simulink model "ModelPrePostNear"  (R2022b)
settings: Solver=FixedStepDiscrete  StartTime=0.0  StopTime=1  RelTol=1e-3  EnableMultiTasking=on
InitFcn:
  | % Initialize model
  | run(['ModelInit.m']);
  | 
  | % load library data
  | GainLibrary_data;
StartFcn:
  | % make sure all the simulated RTC requests are found
  | %RTC_SIM_OBJ.ValidateREQs();
model workspace (MAT data in the model file):
  PreampVolumeTable_Idx = Simulink.Signal
  PreampVolumeTable_Idx.DataType = 'auto'
  PreampVolumeTable_Idx.Dimensions = -1
  PreampVolumeTable_Idx.DimensionsMode = 'auto'
  PreampVolumeTable_Idx.Complexity = 'auto'
  PreampVolumeTable_Idx.SampleTime = -1
  PreampVolumeTable_Idx.SamplingMode = 'auto'
  PreampVolumeTable_Idx.InitialValue = 'uint8([0 255 255 255 255 255])'
  Range = Simulink.Signal
  Range.DataType = 'auto'
  Range.Dimensions = -1
  Range.DimensionsMode = 'auto'
  Range.Complexity = 'auto'
  Range.SampleTime = -1
  Range.SamplingMode = 'auto'
  Table_Idx = Simulink.Signal
  Table_Idx.DataType = 'auto'
  Table_Idx.Dimensions = -1
  Table_Idx.DimensionsMode = 'auto'
  Table_Idx.Complexity = 'auto'
  Table_Idx.SampleTime = -1
  Table_Idx.SamplingMode = 'auto'
undefined symbols (not defined in the file): numAudioIn, preAmp, sys_defs
libraries: FeaturePath x11, RTC x6, SampleRateConverter x4, dspindex x3, EdgePorts x2, ToneBtc x2, dspsrcs4 x2, Router x1, Near1p1Ann x1, EnergyLimiter x1, Limiter x1, Mute x1
settings Model: Creator=kl13806  LastModifiedBy=sc48041
settings SolverCC: AlgebraicLoopSolver=TrustRegion  AutoInsertRateTranBlk=on
settings OptimizationCC: DefaultParameterBehavior=Inlined  DefaultUnderspecifiedDataType=single  EnhancedBackFolding=on  PassReuseOutputArgsAs=Individual arguments  ZeroExternalMemoryAtStartup=off  ZeroInternalMemoryAtStartup=off  MaxStackSize=2048  OptimizeBlockOrder=speed  DifferentSizesBufferReuse=on  OptimizationCustomize=off  EfficientTunableParamExpr=on
settings DebuggingCC: InheritedTsInSrcMsg=none  MultiTaskDSMMsg=none  MultiTaskRateTransMsg=warning  ParameterPrecisionLossMsg=none  ParameterTunabilityLossMsg=error  UnconnectedInputMsg=warning  UnconnectedOutputMsg=warning  UnconnectedLineMsg=warning  BusObjectLabelMismatch=none  UnknownTsInhSupMsg=none  SFUnexpectedBacktrackingDiag=warning  SFNoUnconditionalDefaultTransitionDiag=warning  SFExecutionAtInitializationDiag=none  SFMachineParentedDataDiag=warning  ArithmeticOperatorsInVariantConditions=warning
settings HardwareCC: ProdBitPerPointer=32  ProdBitPerSizeT=32  ProdBitPerPtrDiffT=32  ProdWordSize=32  ProdHWDeviceType=Intel->x86-32 (Windows32)  TargetBitPerPointer=64  TargetBitPerSizeT=64  TargetBitPerPtrDiffT=64  TargetLongLongMode=on  TargetIntDivRoundTo=Zero  TargetEndianess=LittleEndian  TargetWordSize=64  TargetHWDeviceType=MATLAB Host  ProdEqTarget=off
settings ModelReferenceCC: EnableRefExpFcnMdlSchedulingChecks=on
settings SFSimCC: SimUseLocalCustomCode=off  MATLABDynamicMemAlloc=off  CustomCodeUndefinedFunction=UseInterfaceOnly
settings RTWCC: Description=Embedded Coder (host-based shared library target)  SystemTargetFile=ert_shrlib.tlc  GenCodeOnly=on  TemplateMakefile=ert_default_tmf  GenerateReport=on  RetainRTWFile=on  RTWUseLocalCustomCode=off  Toolchain=LCC-win64 v2.4.1 | gmake (64-bit Windows)  IncludeHyperlinkInReport=on  LaunchReport=on  GenerateTraceInfo=on  GenerateTraceReport=on  GenerateTraceReportSl=on  GenerateTraceReportSf=on  GenerateTraceReportEml=on  GenerateCodeMetricsReport=on  GenerateCodeReplacementReport=on
settings CodeAppCC: ForceParamTrailComments=on  IgnoreCustomStorageClasses=off  MaxIdLength=61  OperatorAnnotations=on  SimulinkDataObjDesc=on  SFDataObjDesc=on  InsertBlockDesc=on
settings STFCustomTargetCC: TargetLangStandard=C99 (ISO)  MultiwordLength=256  GenerateSampleERTMain=on  ParMdlRefBuildCompliant=on  CompOptLevelCompliant=on  CombineOutputUpdateFcns=on  ERTCustomFileBanners=on  SupportContinuousTime=off  SupportNonInlinedSFcns=off  RemoveResetFunc=on  SupportVariableSizeSignals=on  MATLABClassNameForMDSCustomization=Simulink.SoftwareTarget.ERTCustomization  ModelStepFunctionPrototypeControlCompliant=on  UseToolchainInfoCompliant=on  SystemTargetFile=ert_shrlib.tlc
settings ERTTargetCC: TargetLangStandard=C99 (ISO)  GenerateSampleERTMain=on  ConcurrentExecutionCompliant=off  SupportVariableSizeSignals=on  CPPClassGenCompliant=off  InlinedParameterPlacement=NonHierarchical  ERTCustomFileTemplate=example_file_process.tlc
settings ConfigComp: CovMetricSettings=dw  CovSaveCumulativeToWorkspaceVar=on  CovSaveSingleToWorkspaceVar=on  CovExternalEMLEnable=off

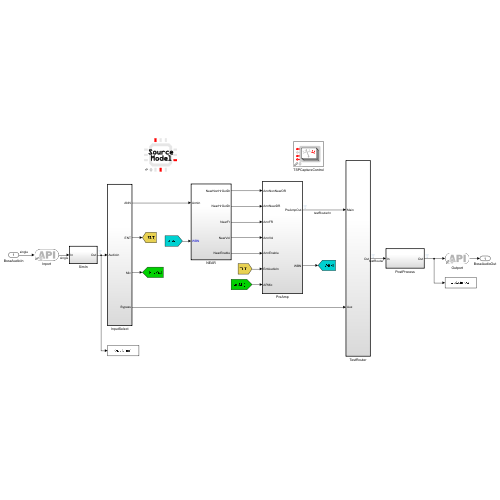
[thumbnail: Simulink's stored preview of the top-level diagram]
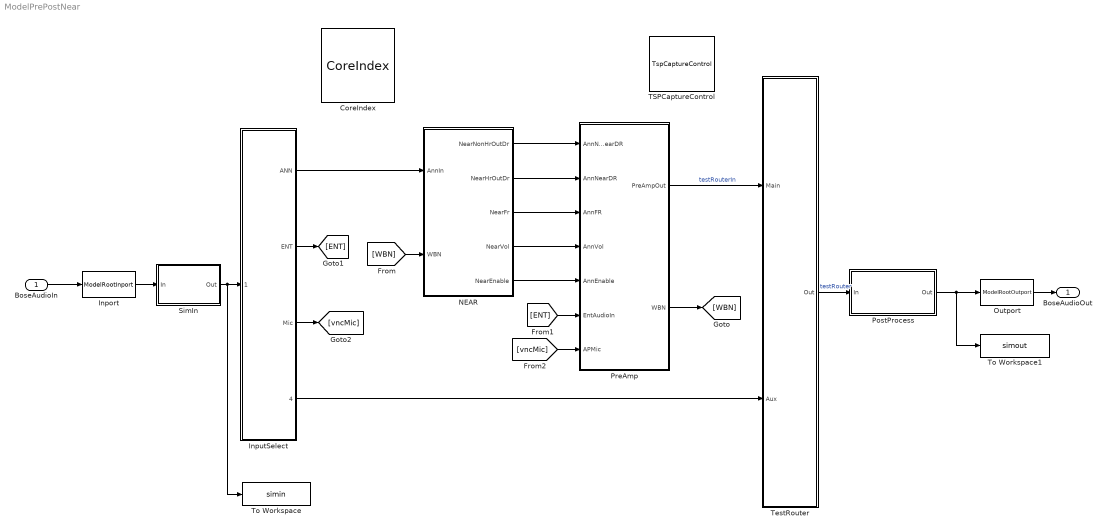
== system ModelPrePostNear ==
  BoseAudioIn : Inport  OutDataTypeStr=single  PortDimensions=[sys_defs.frameSize numAudioIn]  SampleTime=1/sys_defs.Fs * sys_defs.frameSize
  CoreIndex : FeaturePath/CoreIndex  Role=Source Model  CoreIndex=8  Config=[]  AddressingMode=Directly include core number in message identifiers (i.e. simple and static)  CrossCoreApi=None  CrossCoreAllocation=None  CrossCoreSampleTime=-1  BasePeriod=[]  TriggerInit=[-15 -776 80 -679]
      settings: SourceProductName=Bose Talaria
  Inport : EdgePorts/ModelRootInport  Config=ModelRootIn
      settings: SourceProductName=Bose Talaria
  InputSelect : Subsystem  TreatAsAtomicUnit=on
      settings: RTWSystemCode=Nonreusable function
  NEAR : Subsystem  TreatAsAtomicUnit=on
  Outport : EdgePorts/ModelRootOutport  Config=ModelRootOut
      settings: SourceProductName=Bose Talaria
  PostProcess : Subsystem  TreatAsAtomicUnit=on
  PreAmp : Subsystem  TreatAsAtomicUnit=on
  SimIn : Subsystem  TreatAsAtomicUnit=on
  TSPCaptureControl : TSP/TspCaptureControl  TriggerInit=[415 -766 500 -694]
      settings: SourceProductName=Bose Talaria
  TestRouter : Subsystem  TreatAsAtomicUnit=on
  To Workspace : ToWorkspace  VariableName=simin  SampleTime=-1
  To Workspace1 : ToWorkspace  VariableName=simout  SampleTime=-1
  BoseAudioOut : Outport  VectorParamsAs1DForOutWhenUnconnected=off
  wires:
  SimIn/1(Out) -> To Workspace/1, InputSelect/1(AudioIn)
  BoseAudioIn/1 -> Inport/1
  PostProcess/1(Out) -> To Workspace1/1, Outport/1
  TestRouter/1(Out) -> PostProcess/1(In)  "testRouter"
  PreAmp/1(PreAmpOut) -> TestRouter/1(Main)  "testRouterIn"
  InputSelect/4(Bypass) -> TestRouter/2(Aux)
  Inport/1 -> SimIn/1(In)
  Outport/1 -> BoseAudioOut/1
  InputSelect/1(ANN) -> NEAR/1(AnnIn)
  [WBN] -> NEAR/2(WBN)
  NEAR/5(NearEnable) -> PreAmp/5(AnnEnable)
  NEAR/4(NearVol) -> PreAmp/4(AnnVol)
  NEAR/3(NearFr) -> PreAmp/3(AnnFR)
  PreAmp/2(WBN) -> [WBN]
  NEAR/1(NearNonHrOutDr) -> PreAmp/1(AnnNonNearDR)
  NEAR/2(NearHrOutDr) -> PreAmp/2(AnnNearDR)
  InputSelect/2(ENT) -> [ENT]
  [ENT] -> PreAmp/6(EntAudioIn)
  InputSelect/3(Mic) -> [vncMic]
  [vncMic] -> PreAmp/7(APMic)

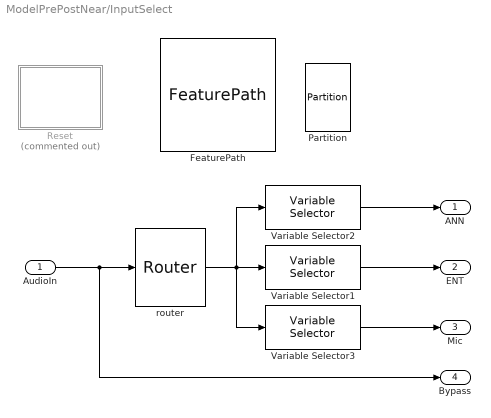
== system ModelPrePostNear/InputSelect ==
  AudioIn : Inport
  FeaturePath : FeaturePath/FeaturePath  FeatureName=InputSelect  IsGroup=on  GroupNumber=0  IsModule=on  TriggerInit=[105 216 220 329]
      settings: SourceProductName=Bose Talaria
  Partition : FeaturePath/Partition  PartitionNumber=0  TriggerInit=[250 241 295 309]
      settings: SourceProductName=Bose Talaria
  Reset : Subsystem  Commented=on
  Variable Selector1 : dspindex/Variable Selector  NumInputs=1  rowsOrCols=Columns  IdxMode=Fixed  Elements=entMap  ZerOneIdxMode=One-based  errmode=Clip Index  FillMode=on  FillValues=0
  Variable Selector2 : dspindex/Variable Selector  NumInputs=1  rowsOrCols=Columns  IdxMode=Fixed  Elements=annMap  ZerOneIdxMode=One-based  errmode=Clip Index  FillMode=on  FillValues=0
  Variable Selector3 : dspindex/Variable Selector  NumInputs=1  rowsOrCols=Columns  IdxMode=Fixed  Elements=vncMic  ZerOneIdxMode=One-based  errmode=Clip Index  FillMode=on  FillValues=0
  router : Router/Router  nInRouterMask=inputSelectChanIn  nOutRouterMask=inputSelectChanOut  outputMapDefaultRouterMask=inputSelectOutputMap
  ANN : Outport
  ENT : Outport  Port=2  VectorParamsAs1DForOutWhenUnconnected=off
  Mic : Outport  Port=3
  Bypass : Outport  Port=4  VectorParamsAs1DForOutWhenUnconnected=off
  wires:
  Variable Selector1/1 -> ENT/1
  AudioIn/1 -> Bypass/1, router/1
  router/1 -> Variable Selector3/1, Variable Selector2/1, Variable Selector1/1
  Variable Selector2/1 -> ANN/1
  Variable Selector3/1 -> Mic/1

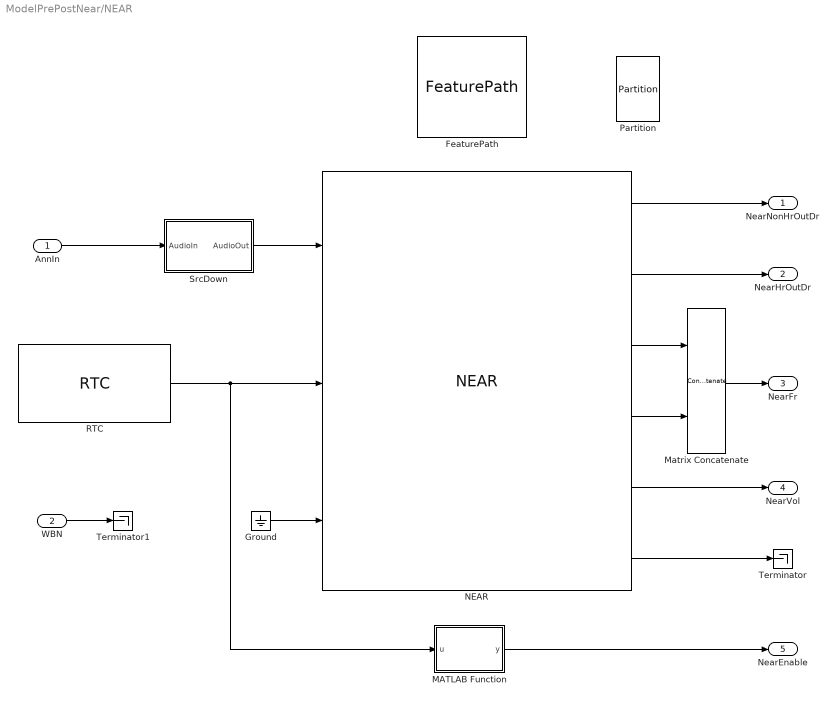
== system ModelPrePostNear/NEAR ==
  AnnIn : Inport
  WBN : Inport  Port=2
  FeaturePath : FeaturePath/FeaturePath  FeatureName=Near  IsGroup=on  GroupNumber=1  IsModule=on  TriggerInit=[15 -306 130 -199]
      settings: SourceProductName=Bose Talaria
  Ground : Ground
  MATLAB Function : MATLAB Function  TreatAsAtomicUnit=on
  Matrix Concatenate : Concatenate  Mode=Multidimensional array  ConcatenateDimension=2
  NEAR : Near1p1Ann/NEAR  near=near
  Partition : FeaturePath/Partition  PartitionNumber=0  TriggerInit=[225 -284 270 -216]
      settings: SourceProductName=Bose Talaria
  RTC : RTC/RTC  REQ_Priority=RTC_Mask.NormalPriority  RequestAtInit=off  EnableRequest=off  REQElemName1=Enable  REQElemType1=uint32  REQElemWidth1=1  REQElemInitial1=[0]  REQElemType2=uint32  REQElemWidth2=1  REQElemInitial2=[]  REQElemType3=uint32  REQElemWidth3=1  REQElemInitial3=[]  REQElemType4=uint32  REQElemWidth4=1  REQElemInitial4=[]  REQElemType5=uint32  REQElemWidth5=1  REQElemInitial5=[]  REQElemType6=uint32  REQElemWidth6=1  REQElemInitial6=[]  REQElemType7=uint32  REQElemWidth7=1  REQElemInitial7=[]  REQElemType8=uint32  REQElemWidth8=1  REQElemInitial8=[]  REQElemType9=uint32  REQElemWidth9=1  REQElemInitial9=[]  REQElemType10=uint32  REQElemWidth10=1  REQElemInitial10=[]  EnableResponse=on  EnableRSP_StatusIn=off  RSPElemType1=uint32  RSPElemWidth1=1  RSPElemType2=uint32  RSPElemWidth2=1  RSPElemType3=uint32  RSPElemWidth3=1  RSPElemType4=uint32  RSPElemWidth4=1  RSPElemType5=uint32  RSPElemWidth5=1  RSPElemType6=uint32  RSPElemWidth6=1  RSPElemType7=uint32  RSPElemWidth7=1  RSPElemType8=uint32  RSPElemWidth8=1  RSPElemType9=uint32  RSPElemWidth9=1  RSPElemType10=uint32  RSPElemWidth10=1  EnableNotification=off  EnableNTF_PrepTrig=off  NTFElemType1=uint32  NTFElemWidth1=1  NTFElemType2=uint32  NTFElemWidth2=1  NTFElemType3=uint32  NTFElemWidth3=1  NTFElemType4=uint32  NTFElemWidth4=1  NTFElemType5=uint32  NTFElemWidth5=1  NTFElemType6=uint32  NTFElemWidth6=1  NTFElemType7=uint32  NTFElemWidth7=1  NTFElemType8=uint32  NTFElemWidth8=1  NTFElemType9=uint32  NTFElemWidth9=1  NTFElemType10=uint32  NTFElemWidth10=1  MaskMessageName=Enable
      settings: SourceProductName=Bose Talaria
  SrcDown : Subsystem  TreatAsAtomicUnit=on
      settings: RTWSystemCode=Nonreusable function
  Terminator : Terminator
  Terminator1 : Terminator
  NearNonHrOutDr : Outport
  NearHrOutDr : Outport  Port=2
  NearFr : Outport  Port=3
  NearVol : Outport  Port=4
  NearEnable : Outport  Port=5
  wires:
  NEAR/1 -> NearNonHrOutDr/1
  AnnIn/1 -> SrcDown/1(AudioIn)
  NEAR/2 -> NearHrOutDr/1
  NEAR/3 -> Matrix Concatenate/1
  NEAR/4 -> Matrix Concatenate/2
  Matrix Concatenate/1 -> NearFr/1
  NEAR/5 -> NearVol/1
  NEAR/6 -> Terminator/1
  RTC/1 -> NEAR/2, MATLAB Function/1(u)
  MATLAB Function/1(y) -> NearEnable/1
  SrcDown/1(AudioOut) -> NEAR/1
  Ground/1 -> NEAR/3
  WBN/1 -> Terminator1/1

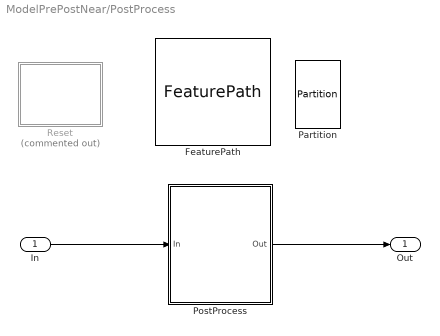
== system ModelPrePostNear/PostProcess ==
  In : Inport
  FeaturePath : FeaturePath/FeaturePath  FeatureName=PostProcess  IsGroup=on  GroupNumber=3  IsModule=on  TriggerInit=[85 -186 200 -79]
      settings: SourceProductName=Bose Talaria
  Partition : FeaturePath/Partition  PartitionNumber=0  TriggerInit=[225 -164 270 -96]
      settings: SourceProductName=Bose Talaria
  PostProcess : Subsystem  TreatAsAtomicUnit=on
      settings: RTWSystemCode=Nonreusable function  RTWFcnNameOpts=Use subsystem name  RTWFileNameOpts=Use subsystem name  FunctionWithSeparateData=on
  Reset : Subsystem  Commented=on
  Out : Outport  VectorParamsAs1DForOutWhenUnconnected=off
  wires:
  In/1 -> PostProcess/1(In)
  PostProcess/1(Out) -> Out/1

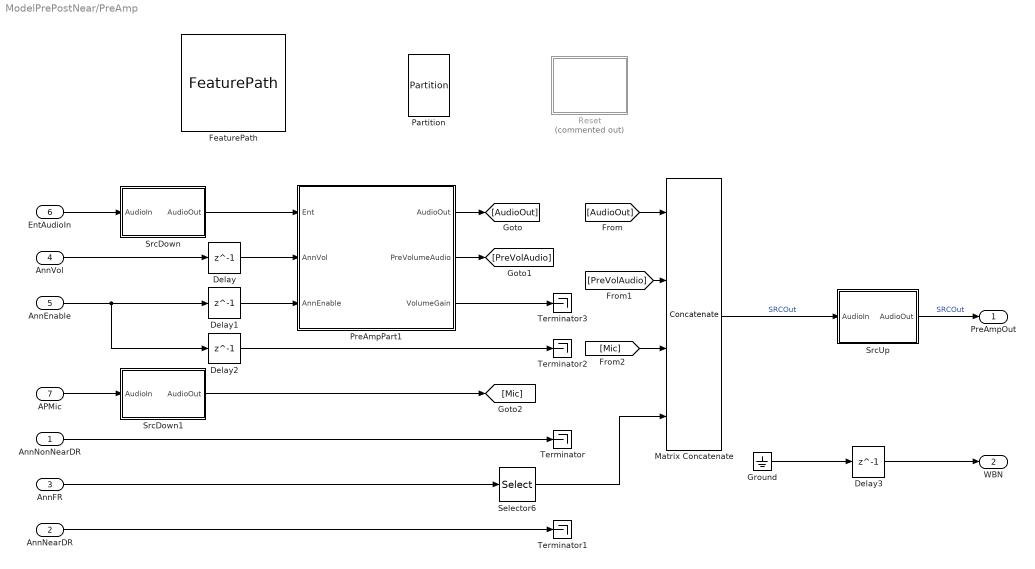
== system ModelPrePostNear/PreAmp ==
  AnnNonNearDR : Inport
  AnnNearDR : Inport  Port=2
  AnnFR : Inport  Port=3
  AnnVol : Inport  Port=4
  AnnEnable : Inport  Port=5
  EntAudioIn : Inport  Port=6
  APMic : Inport  Port=7
  Delay{,1..3} (4 alike) : Delay  DelayLength=1
  FeaturePath : FeaturePath/FeaturePath  FeatureName=PreAmp  IsGroup=on  GroupNumber=2  IsModule=on  TriggerInit=[-135 -246 -20 -139]
      settings: SourceProductName=Bose Talaria
  Ground : Ground
  Matrix Concatenate : Concatenate  NumInputs=4  Mode=Multidimensional array  ConcatenateDimension=2
  Partition : FeaturePath/Partition  PartitionNumber=0  TriggerInit=[115 -224 160 -156]
      settings: SourceProductName=Bose Talaria
  PreAmpPart1 : Subsystem  TreatAsAtomicUnit=on
      settings: RTWSystemCode=Nonreusable function
  Reset : Subsystem  Commented=on
  Selector6 : Selector  NumberOfDimensions=2  InputPortWidth=3  IndexOptions=Select all,Index vector (dialog)  Indices=4,1:19  OutputSizes=1,1
  SrcDown : Subsystem  TreatAsAtomicUnit=on
      settings: RTWSystemCode=Nonreusable function
  SrcDown1 : Subsystem  TreatAsAtomicUnit=on
      settings: RTWSystemCode=Nonreusable function
  SrcUp : Subsystem  TreatAsAtomicUnit=on
      settings: RTWSystemCode=Nonreusable function
  Terminator{,1..3} (4 alike) : Terminator
  PreAmpOut : Outport  VectorParamsAs1DForOutWhenUnconnected=off
  WBN : Outport  Port=2
  wires:
  EntAudioIn/1 -> SrcDown/1(AudioIn)
  Matrix Concatenate/1 -> SrcUp/1(AudioIn)  "SRCOut"
  SrcUp/1(AudioOut) -> PreAmpOut/1  "SRCOut"
  Delay3/1 -> WBN/1
  SrcDown/1(AudioOut) -> PreAmpPart1/1(Ent)
  AnnVol/1 -> Delay/1
  AnnEnable/1 -> Delay2/1, Delay1/1
  Delay/1 -> PreAmpPart1/2(AnnVol)
  Delay1/1 -> PreAmpPart1/3(AnnEnable)
  AnnNonNearDR/1 -> Terminator/1
  AnnNearDR/1 -> Terminator1/1
  AnnFR/1 -> Selector6/1
  APMic/1 -> SrcDown1/1(AudioIn)
  PreAmpPart1/3(VolumeGain) -> Terminator3/1
  Delay2/1 -> Terminator2/1
  Ground/1 -> Delay3/1
  SrcDown1/1(AudioOut) -> [Mic]
  PreAmpPart1/1(AudioOut) -> [AudioOut]
  PreAmpPart1/2(PreVolumeAudio) -> [PreVolAudio]
  [AudioOut] -> Matrix Concatenate/1
  [PreVolAudio] -> Matrix Concatenate/2
  [Mic] -> Matrix Concatenate/3
  Selector6/1 -> Matrix Concatenate/4

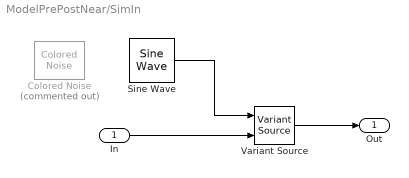
== system ModelPrePostNear/SimIn ==
  In : Inport  OutDataTypeStr=single  SampleTime=1/sys_defs.Fs * sys_defs.frameSize
  Colored Noise : dspsrcs4/Colored Noise  Commented=on  Color=pink  InverseFrequencyPower=1  BoundedOutput=on  NumChannels=2  OutputDataType=single  SamplesPerFrame=32  SampleTime=1/48000  RandomStream=mt19937ar with seed  Seed=67  SimulateUsing=Interpreted execution
  Sine Wave : dspsrcs4/Sine Wave  Amplitude=[0.99*ones(1,numAudioIn)]  Frequency=[150 225 200 275 325]  Phase=zeros(1,numAudioIn)  SampleMode=Discrete  OutComplex=Real  CompMethod=Trigonometric fcn  TableSize=Speed  SampleTime=1/sys_defs.Fs  SamplesPerFrame=sys_defs.frameSize  ResetState=Restart at time zero  OutputFrames=off  dataType=single  wordLen=16  udDataType=sfix(16)  fracBitsMode=Best precision  numFracBits=15  OutDataTypeStr=single  LastOutDataTypeStr=single
  Variant Source : VariantSource  VariantControlMode=sim codegen switching  ShowConditionOnBlock=on
  Out : Outport  VectorParamsAs1DForOutWhenUnconnected=off
  wires:
  In/1 -> Variant Source/2
  Variant Source/1 -> Out/1
  Sine Wave/1 -> Variant Source/1

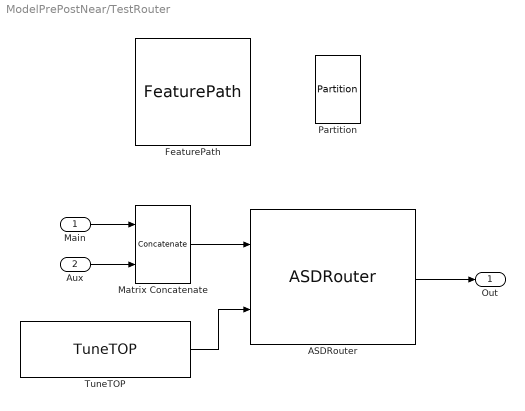
== system ModelPrePostNear/TestRouter ==
  Main : Inport
  Aux : Inport  Port=2
  ASDRouter : ASDRouter/ASDRouter  frameSize=sys_defs.frameSize  nChanOut=sys_defs.nAudioOut  mainSelect=main_select_test  numMainCh=num_main_chs  mainGain=main_gain_test  enableAux=enableAuxTestFlag  numAux=numAuxTestChannels  auxGain=aux_gain_test
  FeaturePath : FeaturePath/FeaturePath  FeatureName=TestRouter  IsGroup=on  GroupNumber=5  IsModule=off  TriggerInit=[290 -166 405 -59]
      settings: SourceProductName=Bose Talaria
  Matrix Concatenate : Concatenate  Mode=Multidimensional array  ConcatenateDimension=2
  Partition : FeaturePath/Partition  PartitionNumber=0  TriggerInit=[470 -149 515 -81]
      settings: SourceProductName=Bose Talaria
  TuneTOP : TuneVar/TuneTOP  TriggerInit=[175 117 345 173]  TopName=AuxSelect  TuneName=AuxSelect  DataType=int32  TunabilityNumber=1  MinValue=[]  MaxValue=[]  BankNumber=0  PreOverlay=false  PostOverlay=false  UseSameName=on  MaskValue=aux_select_test
      settings: SourceProductName=Bose Talaria
  Out : Outport
  wires:
  ASDRouter/1 -> Out/1
  TuneTOP/1 -> ASDRouter/2
  Matrix Concatenate/1 -> ASDRouter/1
  Main/1 -> Matrix Concatenate/1
  Aux/1 -> Matrix Concatenate/2

== system ModelPrePostNear/InputSelect/Reset ==
  MATLAB Function : MATLAB Function  TreatAsAtomicUnit=on
  RTC : RTC/RTC  REQ_Priority=RTC_Mask.NormalPriority  RequestAtInit=off  EnableRequest=on  REQElemType1=uint32  REQElemWidth1=1  REQElemInitial1=[]  REQElemType2=uint32  REQElemWidth2=1  REQElemInitial2=[]  REQElemType3=uint32  REQElemWidth3=1  REQElemInitial3=[]  REQElemType4=uint32  REQElemWidth4=1  REQElemInitial4=[]  REQElemType5=uint32  REQElemWidth5=1  REQElemInitial5=[]  REQElemType6=uint32  REQElemWidth6=1  REQElemInitial6=[]  REQElemType7=uint32  REQElemWidth7=1  REQElemInitial7=[]  REQElemType8=uint32  REQElemWidth8=1  REQElemInitial8=[]  REQElemType9=uint32  REQElemWidth9=1  REQElemInitial9=[]  REQElemType10=uint32  REQElemWidth10=1  REQElemInitial10=[]  EnableResponse=on  EnableRSP_StatusIn=off  RSPElemType1=uint32  RSPElemWidth1=1  RSPElemType2=uint32  RSPElemWidth2=1  RSPElemType3=uint32  RSPElemWidth3=1  RSPElemType4=uint32  RSPElemWidth4=1  RSPElemType5=uint32  RSPElemWidth5=1  RSPElemType6=uint32  RSPElemWidth6=1  RSPElemType7=uint32  RSPElemWidth7=1  RSPElemType8=uint32  RSPElemWidth8=1  RSPElemType9=uint32  RSPElemWidth9=1  RSPElemType10=uint32  RSPElemWidth10=1  EnableNotification=off  EnableNTF_PrepTrig=off  NTFElemType1=uint32  NTFElemWidth1=1  NTFElemType2=uint32  NTFElemWidth2=1  NTFElemType3=uint32  NTFElemWidth3=1  NTFElemType4=uint32  NTFElemWidth4=1  NTFElemType5=uint32  NTFElemWidth5=1  NTFElemType6=uint32  NTFElemWidth6=1  NTFElemType7=uint32  NTFElemWidth7=1  NTFElemType8=uint32  NTFElemWidth8=1  NTFElemType9=uint32  NTFElemWidth9=1  NTFElemType10=uint32  NTFElemWidth10=1  MaskMessageName=Reset
      settings: SourceProductName=Bose Talaria
  wires:
  RTC/1 -> MATLAB Function/Trigger

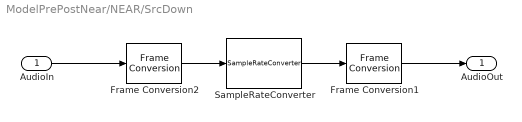
== system ModelPrePostNear/NEAR/SrcDown ==
  AudioIn : Inport
  Frame Conversion1 : FrameConversion  OutFrame=Sample-based
  Frame Conversion2 : FrameConversion
  SampleRateConverter : SampleRateConverter/SampleRateConverter  UPFACTOR=12  DOWNFACTOR=13  OUTFRAME_SIZE=-1  RATE_SELECTOR=Input Sample Rate  FS=48000  FPASSBAND=16500  FHEARING=19000  PASSBAND_RIPPLE=60  STOPBAND_ATTENUATION=60
  AudioOut : Outport
  wires:
  SampleRateConverter/1 -> Frame Conversion1/1
  AudioIn/1 -> Frame Conversion2/1
  Frame Conversion1/1 -> AudioOut/1
  Frame Conversion2/1 -> SampleRateConverter/1

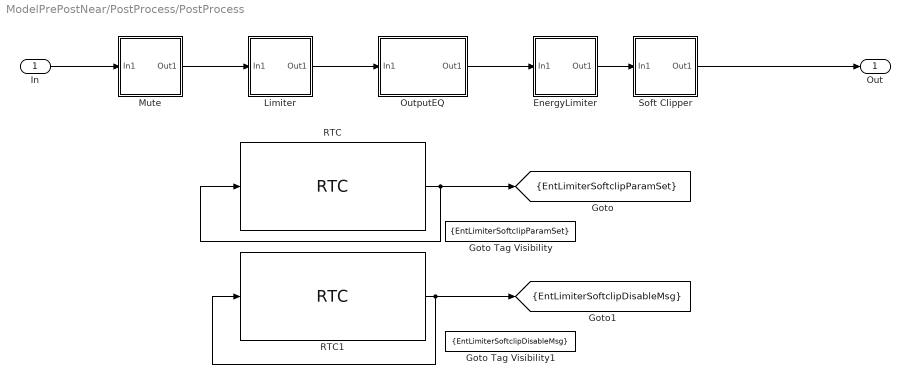
== system ModelPrePostNear/PostProcess/PostProcess ==
  In : Inport
  EnergyLimiter : Subsystem
  Goto Tag Visibility : GotoTagVisibility  GotoTag=EntLimiterSoftclipParamSet
  Goto Tag Visibility1 : GotoTagVisibility  GotoTag=EntLimiterSoftclipDisableMsg
  Limiter : Subsystem
  Mute : Subsystem
  OutputEQ : Subsystem
  RTC : RTC/RTC  Description=|  REQ_Priority=RTC_Mask.NormalPriority  RequestAtInit=off  EnableRequest=off  REQElemName1=paramSet  REQElemType1=uint32  REQElemWidth1=1  REQElemInitial1=1  REQElemType2=uint32  REQElemWidth2=1  REQElemInitial2=[]  REQElemType3=uint32  REQElemWidth3=1  REQElemInitial3=[]  REQElemType4=uint32  REQElemWidth4=1  REQElemInitial4=[]  REQElemType5=uint32  REQElemWidth5=1  REQElemInitial5=[]  REQElemType6=uint32  REQElemWidth6=1  REQElemInitial6=[]  REQElemType7=uint32  REQElemWidth7=1  REQElemInitial7=[]  REQElemType8=uint32  REQElemWidth8=1  REQElemInitial8=[]  REQElemType9=uint32  REQElemWidth9=1  REQElemInitial9=[]  REQElemType10=uint32  REQElemWidth10=1  REQElemInitial10=[]  EnableResponse=on  EnableRSP_StatusIn=off  RSPElemName1=paramSet  RSPElemType1=uint32  RSPElemWidth1=1  RSPElemType2=uint32  RSPElemWidth2=1  RSPElemType3=uint32  RSPElemWidth3=1  RSPElemType4=uint32  RSPElemWidth4=1  RSPElemType5=uint32  RSPElemWidth5=1  RSPElemType6=uint32  RSPElemWidth6=1  RSPElemType7=uint32  RSPElemWidth7=1  RSPElemType8=uint32  RSPElemWidth8=1  RSPElemType9=uint32  RSPElemWidth9=1  RSPElemType10=uint32  RSPElemWidth10=1  EnableNotification=off  EnableNTF_PrepTrig=off  NTFElemType1=uint32  NTFElemWidth1=1  NTFElemType2=uint32  NTFElemWidth2=1  NTFElemType3=uint32  NTFElemWidth3=1  NTFElemType4=uint32  NTFElemWidth4=1  NTFElemType5=uint32  NTFElemWidth5=1  NTFElemType6=uint32  NTFElemWidth6=1  NTFElemType7=uint32  NTFElemWidth7=1  NTFElemType8=uint32  NTFElemWidth8=1  NTFElemType9=uint32  NTFElemWidth9=1  NTFElemType10=uint32  NTFElemWidth10=1  MaskMessageName=LimiterSoftclipParamSet
      | Choose parameter set for limiter and soft clipper.
      | 1: normal set
      | 2: used in start-stop situation
      settings: SourceProductName=Bose Talaria
  RTC1 : RTC/RTC  REQ_Priority=RTC_Mask.NormalPriority  RequestAtInit=off  EnableRequest=off  REQElemName1=disableMsg  REQElemType1=uint32  REQElemWidth1=1  REQElemInitial1=0  REQElemType2=uint32  REQElemWidth2=1  REQElemInitial2=[]  REQElemType3=uint32  REQElemWidth3=1  REQElemInitial3=[]  REQElemType4=uint32  REQElemWidth4=1  REQElemInitial4=[]  REQElemType5=uint32  REQElemWidth5=1  REQElemInitial5=[]  REQElemType6=uint32  REQElemWidth6=1  REQElemInitial6=[]  REQElemType7=uint32  REQElemWidth7=1  REQElemInitial7=[]  REQElemType8=uint32  REQElemWidth8=1  REQElemInitial8=[]  REQElemType9=uint32  REQElemWidth9=1  REQElemInitial9=[]  REQElemType10=uint32  REQElemWidth10=1  REQElemInitial10=[]  EnableResponse=on  EnableRSP_StatusIn=off  RSPElemName1=disableMsg  RSPElemType1=uint32  RSPElemWidth1=1  RSPElemType2=uint32  RSPElemWidth2=1  RSPElemType3=uint32  RSPElemWidth3=1  RSPElemType4=uint32  RSPElemWidth4=1  RSPElemType5=uint32  RSPElemWidth5=1  RSPElemType6=uint32  RSPElemWidth6=1  RSPElemType7=uint32  RSPElemWidth7=1  RSPElemType8=uint32  RSPElemWidth8=1  RSPElemType9=uint32  RSPElemWidth9=1  RSPElemType10=uint32  RSPElemWidth10=1  EnableNotification=off  EnableNTF_PrepTrig=off  NTFElemType1=uint32  NTFElemWidth1=1  NTFElemType2=uint32  NTFElemWidth2=1  NTFElemType3=uint32  NTFElemWidth3=1  NTFElemType4=uint32  NTFElemWidth4=1  NTFElemType5=uint32  NTFElemWidth5=1  NTFElemType6=uint32  NTFElemWidth6=1  NTFElemType7=uint32  NTFElemWidth7=1  NTFElemType8=uint32  NTFElemWidth8=1  NTFElemType9=uint32  NTFElemWidth9=1  NTFElemType10=uint32  NTFElemWidth10=1  MaskMessageName=LimiterSoftclipDisable
      settings: SourceProductName=Bose Talaria
  Soft Clipper : Subsystem
  Out : Outport  VectorParamsAs1DForOutWhenUnconnected=off
  tag scope: EntLimiterSoftclipDisableMsg=scoped, EntLimiterSoftclipParamSet=scoped
  wires:
  Mute/1(Out1) -> Limiter/1(In1)
  Limiter/1(Out1) -> OutputEQ/1(In1)
  In/1 -> Mute/1(In1)
  OutputEQ/1(Out1) -> EnergyLimiter/1(In1)
  EnergyLimiter/1(Out1) -> Soft Clipper/1(In1)
  RTC1/1 -> RTC1/1, [EntLimiterSoftclipDisableMsg]
  RTC/1 -> RTC/1, [EntLimiterSoftclipParamSet]
  Soft Clipper/1(Out1) -> Out/1

== system ModelPrePostNear/PostProcess/Reset ==
  MATLAB Function : MATLAB Function  TreatAsAtomicUnit=on
  RTC : RTC/RTC  REQ_Priority=RTC_Mask.NormalPriority  RequestAtInit=off  EnableRequest=on  REQElemType1=uint32  REQElemWidth1=1  REQElemInitial1=[]  REQElemType2=uint32  REQElemWidth2=1  REQElemInitial2=[]  REQElemType3=uint32  REQElemWidth3=1  REQElemInitial3=[]  REQElemType4=uint32  REQElemWidth4=1  REQElemInitial4=[]  REQElemType5=uint32  REQElemWidth5=1  REQElemInitial5=[]  REQElemType6=uint32  REQElemWidth6=1  REQElemInitial6=[]  REQElemType7=uint32  REQElemWidth7=1  REQElemInitial7=[]  REQElemType8=uint32  REQElemWidth8=1  REQElemInitial8=[]  REQElemType9=uint32  REQElemWidth9=1  REQElemInitial9=[]  REQElemType10=uint32  REQElemWidth10=1  REQElemInitial10=[]  EnableResponse=on  EnableRSP_StatusIn=off  RSPElemType1=uint32  RSPElemWidth1=1  RSPElemType2=uint32  RSPElemWidth2=1  RSPElemType3=uint32  RSPElemWidth3=1  RSPElemType4=uint32  RSPElemWidth4=1  RSPElemType5=uint32  RSPElemWidth5=1  RSPElemType6=uint32  RSPElemWidth6=1  RSPElemType7=uint32  RSPElemWidth7=1  RSPElemType8=uint32  RSPElemWidth8=1  RSPElemType9=uint32  RSPElemWidth9=1  RSPElemType10=uint32  RSPElemWidth10=1  EnableNotification=off  EnableNTF_PrepTrig=off  NTFElemType1=uint32  NTFElemWidth1=1  NTFElemType2=uint32  NTFElemWidth2=1  NTFElemType3=uint32  NTFElemWidth3=1  NTFElemType4=uint32  NTFElemWidth4=1  NTFElemType5=uint32  NTFElemWidth5=1  NTFElemType6=uint32  NTFElemWidth6=1  NTFElemType7=uint32  NTFElemWidth7=1  NTFElemType8=uint32  NTFElemWidth8=1  NTFElemType9=uint32  NTFElemWidth9=1  NTFElemType10=uint32  NTFElemWidth10=1  MaskMessageName=Reset
      settings: SourceProductName=Bose Talaria
  wires:
  RTC/1 -> MATLAB Function/Trigger

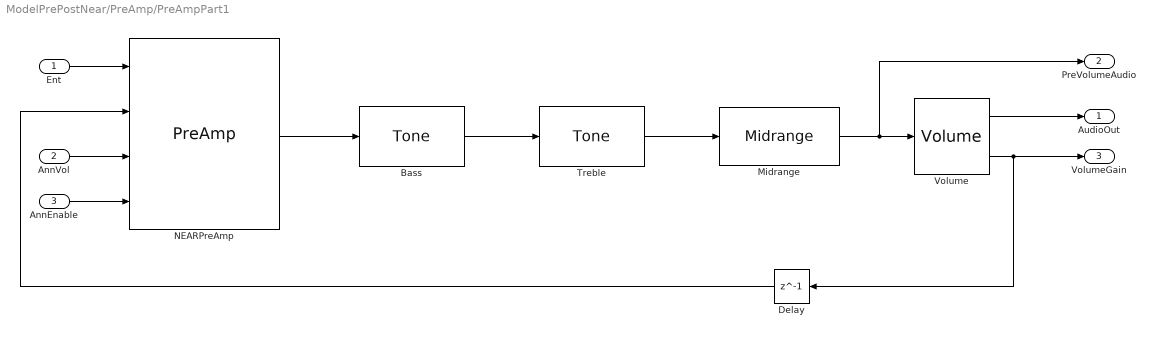
== system ModelPrePostNear/PreAmp/PreAmpPart1 ==
  Ent : Inport
  AnnVol : Inport  Port=2
  AnnEnable : Inport  Port=3
  Bass : ToneBtc/Tone  FeatureName=Bass  Config=[]  TriggerInit=[215 80 320 140]
      settings: SourceProductName=Bose Blocklib
  Delay : Delay  DelayLength=1
  Midrange : MidrangeBtc/Midrange  FeatureName=Midrange  Config=[]
      settings: SourceProductName=Bose Blocklib
  NEARPreAmp : PreAmpLib/PreAmp  Config=[preAmp]
  Treble : ToneBtc/Tone  FeatureName=Treble  Config=[]  TriggerInit=[395 80 500 140]
      settings: SourceProductName=Bose Blocklib
  Volume : VolumeBtc/Volume  FeatureName=Volume  Config=Volume  EnableGainOut=on  TriggerInit=[770 72 845 148]
      settings: SourceProductName=Bose Blocklib
  AudioOut : Outport
  PreVolumeAudio : Outport  Port=2
  VolumeGain : Outport  Port=3
  wires:
  Ent/1 -> NEARPreAmp/1
  Bass/1 -> Treble/1
  Treble/1 -> Midrange/1
  Midrange/1 -> PreVolumeAudio/1, Volume/1
  Volume/1 -> AudioOut/1
  Volume/2 -> Delay/1, VolumeGain/1
  NEARPreAmp/1 -> Bass/1
  Delay/1 -> NEARPreAmp/2
  AnnVol/1 -> NEARPreAmp/3
  AnnEnable/1 -> NEARPreAmp/4

== system ModelPrePostNear/PreAmp/Reset ==
  MATLAB Function : MATLAB Function  TreatAsAtomicUnit=on
  RTC : RTC/RTC  REQ_Priority=RTC_Mask.NormalPriority  RequestAtInit=off  EnableRequest=on  REQElemType1=uint32  REQElemWidth1=1  REQElemInitial1=[]  REQElemType2=uint32  REQElemWidth2=1  REQElemInitial2=[]  REQElemType3=uint32  REQElemWidth3=1  REQElemInitial3=[]  REQElemType4=uint32  REQElemWidth4=1  REQElemInitial4=[]  REQElemType5=uint32  REQElemWidth5=1  REQElemInitial5=[]  REQElemType6=uint32  REQElemWidth6=1  REQElemInitial6=[]  REQElemType7=uint32  REQElemWidth7=1  REQElemInitial7=[]  REQElemType8=uint32  REQElemWidth8=1  REQElemInitial8=[]  REQElemType9=uint32  REQElemWidth9=1  REQElemInitial9=[]  REQElemType10=uint32  REQElemWidth10=1  REQElemInitial10=[]  EnableResponse=on  EnableRSP_StatusIn=off  RSPElemType1=uint32  RSPElemWidth1=1  RSPElemType2=uint32  RSPElemWidth2=1  RSPElemType3=uint32  RSPElemWidth3=1  RSPElemType4=uint32  RSPElemWidth4=1  RSPElemType5=uint32  RSPElemWidth5=1  RSPElemType6=uint32  RSPElemWidth6=1  RSPElemType7=uint32  RSPElemWidth7=1  RSPElemType8=uint32  RSPElemWidth8=1  RSPElemType9=uint32  RSPElemWidth9=1  RSPElemType10=uint32  RSPElemWidth10=1  EnableNotification=off  EnableNTF_PrepTrig=off  NTFElemType1=uint32  NTFElemWidth1=1  NTFElemType2=uint32  NTFElemWidth2=1  NTFElemType3=uint32  NTFElemWidth3=1  NTFElemType4=uint32  NTFElemWidth4=1  NTFElemType5=uint32  NTFElemWidth5=1  NTFElemType6=uint32  NTFElemWidth6=1  NTFElemType7=uint32  NTFElemWidth7=1  NTFElemType8=uint32  NTFElemWidth8=1  NTFElemType9=uint32  NTFElemWidth9=1  NTFElemType10=uint32  NTFElemWidth10=1  MaskMessageName=Reset
      settings: SourceProductName=Bose Talaria
  wires:
  RTC/1 -> MATLAB Function/Trigger

== system ModelPrePostNear/PreAmp/SrcDown ==
  AudioIn : Inport
  Frame Conversion1 : FrameConversion  OutFrame=Sample-based
  Frame Conversion2 : FrameConversion
  SampleRateConverter : SampleRateConverter/SampleRateConverter  UPFACTOR=12  DOWNFACTOR=13  OUTFRAME_SIZE=-1  RATE_SELECTOR=Input Sample Rate  FS=48000  FPASSBAND=16500  FHEARING=19000  PASSBAND_RIPPLE=60  STOPBAND_ATTENUATION=60
  AudioOut : Outport
  wires:
  SampleRateConverter/1 -> Frame Conversion1/1
  AudioIn/1 -> Frame Conversion2/1
  Frame Conversion1/1 -> AudioOut/1
  Frame Conversion2/1 -> SampleRateConverter/1

== system ModelPrePostNear/PreAmp/SrcDown1 ==
  AudioIn : Inport
  Frame Conversion1 : FrameConversion  OutFrame=Sample-based
  Frame Conversion2 : FrameConversion
  SampleRateConverter : SampleRateConverter/SampleRateConverter  UPFACTOR=12  DOWNFACTOR=13  OUTFRAME_SIZE=-1  RATE_SELECTOR=Input Sample Rate  FS=48000  FPASSBAND=16500  FHEARING=19000  PASSBAND_RIPPLE=60  STOPBAND_ATTENUATION=60
  AudioOut : Outport
  wires:
  SampleRateConverter/1 -> Frame Conversion1/1
  AudioIn/1 -> Frame Conversion2/1
  Frame Conversion1/1 -> AudioOut/1
  Frame Conversion2/1 -> SampleRateConverter/1

== system ModelPrePostNear/PreAmp/SrcUp ==
  AudioIn : Inport
  Frame Conversion : FrameConversion
  Frame Conversion1 : FrameConversion  OutFrame=Sample-based
  SampleRateConverter1 : SampleRateConverter/SampleRateConverter  UPFACTOR=13  DOWNFACTOR=12  OUTFRAME_SIZE=-1  RATE_SELECTOR=Input Sample Rate  FS=48000  FPASSBAND=16500  FHEARING=19000  PASSBAND_RIPPLE=60  STOPBAND_ATTENUATION=60
  AudioOut : Outport
  wires:
  SampleRateConverter1/1 -> Frame Conversion1/1
  Frame Conversion/1 -> SampleRateConverter1/1
  Frame Conversion1/1 -> AudioOut/1
  AudioIn/1 -> Frame Conversion/1

== system ModelPrePostNear/PostProcess/PostProcess/EnergyLimiter ==
  In1 : Inport
  EnergyLimiter : EnergyLimiter/EnergyLimiter  EnableGainLimiter=EnableGainLimiter  EnergyMeasurementTimeConstantInSeconds=EnergyMeasurementTimeConstantInSeconds  GainChangeStepIndB=GainChangeStepIndB  MaxEnergyLevelIndB=MaxEnergyLevelIndB  EnergyAdjustmentFactorIndB=EnergyAdjustmentFactorIndB  MaxChannels=MaxChannels  GainIncreaseDurationInSeconds=GainIncreaseDurationInSeconds  GainDecreaseDurationInSeconds=GainDecreaseDurationInSeconds  MaxGainReductionIndB=MaxGainReductionIndB  sample_rate_in_hertz=sample_rate_in_hertz  frameSize=frameSize  CurrentGainVal=CurrentGainVal
  Terminator : Terminator
  Out1 : Outport
  wires:
  EnergyLimiter/2 -> Terminator/1
  In1/1 -> EnergyLimiter/1
  EnergyLimiter/1 -> Out1/1

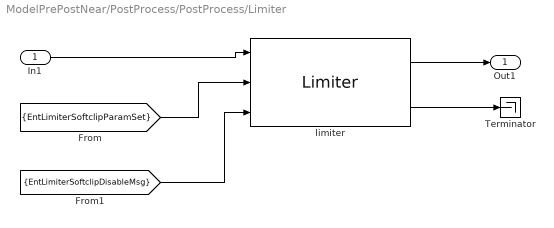
== system ModelPrePostNear/PostProcess/PostProcess/Limiter ==
  In1 : Inport
  Terminator : Terminator
  limiter : Limiter/Limiter  attackDB=10e3 * ones(1,sys_defs.number_of_output_audio_channels)  decayDB=100 * ones(1,sys_defs.number_of_output_audio_channels)  maxAttackTuningValue=10 * ones(1,sys_defs.number_of_output_audio_channels)  threshold=0.9 * ones(1,sys_defs.number_of_output_audio_channels)  attackDB_low=10e3 * ones(1,sys_defs.number_of_output_audio_channels)  decayDB_low=100 * ones(1,sys_defs.number_of_output_audio_channels)  maxAttack_low=10 * ones(1,sys_defs.number_of_output_audio_channels)  threshold_low=0.9 * ones(1,sys_defs.number_of_output_audio_channels)
  Out1 : Outport  VectorParamsAs1DForOutWhenUnconnected=off
  wires:
  In1/1 -> limiter/1
  limiter/1 -> Out1/1
  [EntLimiterSoftclipParamSet] -> limiter/2
  [EntLimiterSoftclipDisableMsg] -> limiter/3
  limiter/2 -> Terminator/1

== system ModelPrePostNear/PostProcess/PostProcess/Mute ==
  In1 : Inport
  mute : Mute/mute  initial_mute_state=ent_mute_init  samplesPerFrame=32  MaskFeatureName=Mute
  Out1 : Outport  VectorParamsAs1DForOutWhenUnconnected=off
  wires:
  In1/1 -> mute/1
  mute/1 -> Out1/1

== system ModelPrePostNear/PostProcess/PostProcess/OutputEQ ==
  In1 : Inport
  Pooliir with Non-Trivial Translations : PooliirLib/PooliirwithNonTrivialTranslations  maxNumStages=64  numStages=outputEQ.numStages  sosCoefficients=outputEQ.coeffs  FeatureName=EQ
  Out1 : Outport
  wires:
  Pooliir with Non-Trivial Translations/1 -> Out1/1
  In1/1 -> Pooliir with Non-Trivial Translations/1

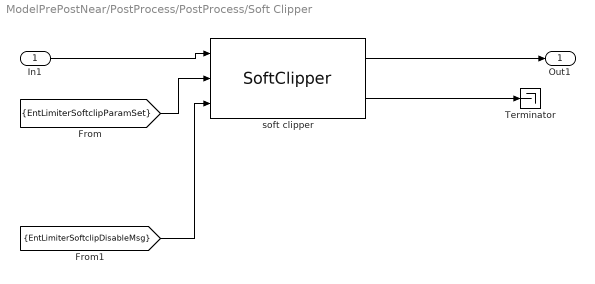
== system ModelPrePostNear/PostProcess/PostProcess/Soft Clipper ==
  In1 : Inport
  Terminator : Terminator
  soft clipper : Softclipper/SoftClipper  MaxXminLow=0.65  MaskXmin=0.65  MaskYMax=1  MaskYMaxLow=1
  Out1 : Outport  VectorParamsAs1DForOutWhenUnconnected=off
  wires:
  In1/1 -> soft clipper/1
  soft clipper/1 -> Out1/1
  [EntLimiterSoftclipParamSet] -> soft clipper/2
  [EntLimiterSoftclipDisableMsg] -> soft clipper/3
  soft clipper/2 -> Terminator/1

== matlab function ModelPrePostNear/PreAmp/Reset/MATLAB Function ==
  events: trigger input FUNCTION_CALL_EVENT
function fcn()

if coder.target('Rtw')
    coder.ceval('Model_Target_DRFDP_initialize');
    coder.ceval('Model_Target_FRFDP_initialize');
    coder.ceval('Model_Target_ExpandTailComponents_initialize');
    coder.ceval('Model_Target_TrebleandSurroundDelays_initialize');
    coder.ceval('Model_Target_Medusa5H1Part3_initialize');
    coder.ceval('Model_Target_Subsystem_initialize');
    
    coder.ceval('Model_Target_PreAmpPart1_Start');
    coder.ceval('Model_Target_SRCIn_Start');
%     coder.ceval('Model_Target_AudioPilot35_Start');
    coder.ceval('Model_Target_Medusa5H1Part1_Start');
    coder.ceval('Model_Target_Medusa5H1Part2_Start');
    coder.ceval('Model_Target_Medusa5H1Part3_Start');

    coder.ceval('Model_Target_PreAmpPart1_Init');
    coder.ceval('Model_Target_PreAmpPart2_Init');
%     coder.ceval('Model_Target_SRCIn_Init');
%     coder.ceval('Model_Target_SRCOut_Init');
%     coder.ceval('Model_Target_AudioPilot35_Init');
    coder.ceval('Model_Target_Medusa5H1Part1_Init');
    coder.ceval('Model_Target_Medusa5H1Part2_Init');
    coder.ceval('Model_Target_Medusa5H1Part3_Init');
end

== matlab function ModelPrePostNear/InputSelect/Reset/MATLAB Function ==
  events: trigger input FUNCTION_CALL_EVENT
function fcn()

if coder.target('Rtw')
    coder.ceval('Model_Target_InputSelect_Init');
end

== matlab function ModelPrePostNear/PostProcess/Reset/MATLAB Function ==
  events: trigger input FUNCTION_CALL_EVENT
function fcn()

if coder.target('Rtw')
    coder.ceval('Model_Target_PostProcess_initialize');
    coder.ceval('Model_Target_PostProcess_Start');
    coder.ceval('Model_Target_PostProcess_Init');
end

== matlab function ModelPrePostNear/NEAR/MATLAB Function ==
  data: u input; y output
function y = fcn(u)

y = u;
